simulink model "Generic_13"  (R2022b)
settings: Solver=VariableStepAuto  StartTime=0.0  StopTime=10.0  RelTol=1e-3
values from neighbouring files (symbols this model uses):
  A = cell2mat(A_cell)    [MPCController1.m]    (also in MPC_Fmincon.m)
  B = cell2mat(B_cell)    [MPCController1.m]    (also in MPC_Fmincon.m)
  brake_select = ones(length(speed), length(steering_angle))    [TwoDLook_uptable.m]
  curvature = 0.000:0.001:1    [TwoDLook_uptable.m]
  m = 1600    [MPCController1.m]    (also in MPCController2.m; MPC_Fmincon.m)
  speed = 0:0.1:100    [TwoDLook_uptable.m]
undefined symbols (not defined in the file or in its folder): Amplifier, DiscIntNeverNeededParam, K_d_yawrate, K_dsteering, k_speed, k_stanley, kd, ki, kp, path_curvature
libraries: CarMaker4SL x121, simulink x12, cstblocks x7, autolibshared x1, mpcadaslib x1
(part 4 of 5)

== matlab function Generic_13/CreateBus VhclCtrl/Stanley  steering & speed//Brake controller/Road sensor set & path planning/Road sensor set & path planning/Cross_track_error_calcuation/Cross_track_error_calcuation ==
  data: x_vehicle input; cte output; y_vehicle input; x_point input; y_point input; denominator output; x2 input; y2 input
function [cte,denominator]= calculate_cross_track_error(x_vehicle, y_vehicle, x_point, y_point,x2,y2)
    % Calculate cross-track error for a given vehicle position and single point
    function cte = calculate_perpendicular_distance(x_vehicle, y_vehicle, x_point, y_point)
    % Calculate the perpendicular distance from the vehicle to the point

    % Coordinates of the point
    x1 = x_point;
    y1 = y_point;
    %x2 = x_vehicle;
    %y2 = y_vehicle;

    % Calculate the cross-track error using the formula for the distance from a point to a line
    numerator = (x2 - x1) * (y1 - y_vehicle) - (x1 - x_vehicle) * (y2 - y1);
    denominator = sqrt((x2 - x1)^2 + (y2 - y1)^2);

    % Ensure that the denominator is not zero to avoid division by zero
    if denominator ~= 0
        cte = (numerator / denominator);
    else
        cte = 0;
    end
end
    % Calculate cross-track error as the perpendicular distance
    cte = calculate_perpendicular_distance(x_vehicle, y_vehicle, x_point, y_point);
end

== matlab function Generic_13/CreateBus VhclCtrl/Stanley  steering & speed//Brake controller/Road sensor set & path planning/Road sensor set & path planning/path_planning/Basic_obstacle avoidance ==
  data: Car_x input; updated_path output; Car_y input; dx input; dy input; object_width input; object_length input; path_x input; path_y input; car_v input; car_v_ceil input
function updated_path = obstacleAvoidanceSimulink(Car_x, Car_y, dx, dy, object_width, object_length, path_x, path_y,car_v, car_v_ceil)
    % Parameters
    if car_v >14
    safety_distance = car_v; % Adjust based on your requirements
    else
        safety_distance = 14;
    end
    %disp(car_v)
    % Check if the vehicle is close to the object
    distance_to_object = sqrt(dx^2 + dy^2);
    if (distance_to_object-object_length < safety_distance && distance_to_object > 0) && dx>0
        % Calculate the trajectory to avoid the entire obstacle
        angle_to_object = atan2(dy, dx);
        object_heading = atan2(object_length, object_width); % Assuming object is aligned with x-axis

        % Calculate new position to avoid the entire obstacle
        new_x = -1*(path_x + (car_v_ceil + object_length) * sin(angle_to_object + object_heading));
        new_y = -1*(path_y + (car_v_ceil + object_width/2) * cos(angle_to_object + object_heading));

        % Update the path to follow the new trajectory
        updated_path = [new_x; new_y] * ones(1, length(path_x));
    else
        updated_path = [path_x; path_y];
        %window_size = 5; % adjust the window size as needed
    %path_curvature = smoothdata(path_curvature, 'movmean', window_size)
    end
end

== matlab function Generic_13/CreateBus VhclCtrl/Stanley  steering & speed//Brake controller/Stanley_controller_with_thottle_and_brake_commands/MPCLongitudianl_contorl/MATLAB Function1 ==
  data: speed input; desired_speed output; distance_to_obstacle input; min_speed input
function desired_speed = advancedCollisionAvoidance(speed, distance_to_obstacle, min_speed)
    % Parameters
    max_acceleration = 3.0; % Maximum allowable acceleration
    max_deceleration = 5.0; % Maximum allowable deceleration
    prediction_horizon = 5; % Prediction horizon in seconds
    time_step = 0.1; % Time step for prediction
    safety_factor = 1.2; % Safety factor for braking distance estimation
    function braking_distance = calculateBrakingDistance(speed, max_deceleration, safety_factor)
    % Estimate the braking distance
    braking_distance = (speed^2) / (2 * max_deceleration) * safety_factor;
    end
    % Calculate the remaining braking distance
    braking_distance = calculateBrakingDistance(speed, max_deceleration, safety_factor);

    % Create a prediction model (simple linear model)
    A = 1; % State transition matrix
    B = -1; % Input matrix
    C = 1; % Output matrix
    Q = 1; % State cost
    R = 1; % Input cost
    N = 5; % Prediction horizon
    
    % Formulate the quadratic cost function
    H = blkdiag(2*(Q + R), repmat(2*Q, 1, N-1));
    
    % Constraints
    lb = min_speed * ones(N, 1);
    ub = speed * ones(N, 1) + max_acceleration * prediction_horizon * time_step;
    
    % Formulate the inequality constraints
    A_ineq = [eye(N); -eye(N)];
    b_ineq = [ub; -lb];
    
    % Initial guess (simple constant acceleration)
    u0 = ones(N, 1) * max_acceleration;
    
    % Solve the quadratic program
    options = optimoptions('quadprog', 'Display', 'off');
    u = quadprog(H, [], A_ineq, b_ineq, [], [], lb, ub, u0, options);
    
    % Apply the first control input as the desired acceleration
    desired_acceleration = u(1);
    
    % Adjust acceleration based on the distance to the obstacle and remaining braking distance
    if distance_to_obstacle < braking_distance
        % Apply maximum deceleration to stop before the obstacle
        desired_acceleration = -max_deceleration;
    end
    
    % Update the speed using the dynamics model
    desired_speed = speed + desired_acceleration * time_step;
    
    % Ensure the desired speed is within limits
    desired_speed = max(min_speed, min(desired_speed, speed + max_deceleration * time_step));
end

== matlab function Generic_13/CreateBus VhclCtrl/Stanley  steering & speed//Brake controller/Stanley_controller_with_thottle_and_brake_commands/MPCLongitudianl_contorl/Speed_regulator/Desired_speed_calc ==
  data: current_speed input; desired_speed output; distance_to_obstacle input; braking_distance input; relative_velocity input; speed_to_reach input; min_speed input; closing_velocity output; effective_distance output; safe_following_distance output
function [desired_speed,closing_velocity,effective_distance,safe_following_distance]= advancedCollisionAvoidance(current_speed, distance_to_obstacle,braking_distance, relative_velocity, speed_to_reach, min_speed)
    

    % Parameters
    max_deceleration = 5.0; % Maximum deceleration (adjust based on your requirements)
    reaction_time = 1.0; % Reaction time of the driver (adjust based on your requirements)
    % Calculate the remaining braking distance
    %braking_distance = calculateBrakingDistance(current_speed, max_deceleration, safety_factor);
    % Calculate the time required to stop the vehicle
    time_to_stop = current_speed / max_deceleration;

    % Calculate the required deceleration to stop before the obstacle
    required_deceleration = -current_speed / time_to_stop;

    % Calculate the projected distance the vehicle would cover during reaction time
    reaction_distance = current_speed * reaction_time;

    % Calculate the safe following distance based on reaction time and braking distance
    safe_following_distance = reaction_distance + braking_distance;

    % Calculate the effective distance to the obstacle considering reaction time
    effective_distance = distance_to_obstacle - reaction_distance;

    % Calculate the relative closing velocity
    closing_velocity = current_speed ;%- relative_velocity;

    % Determine if collision is imminent and adjust speed accordingly
    if (effective_distance < safe_following_distance-current_speed-5 && closing_velocity > 0)&& distance_to_obstacle ~=0
        % Apply maximum deceleration to avoid collision
        desired_speed = max(min_speed, current_speed + required_deceleration);
    elseif distance_to_obstacle>0 && distance_to_obstacle <5 && current_speed > 0
        desired_speed = 0;
    else
        desired_speed = speed_to_reach;
    end
end

== matlab function Generic_13/CreateBus VhclCtrl/Stanley  steering & speed//Brake controller/Stanley_controller_with_thottle_and_brake_commands/MPCLongitudianl_contorl/Speed_regulator/status_changing ==
  data: current_speed input; braking output; distance_to_obstacle input; relative_velocity input; steering_angle input; steering output; resume_driving output
function [braking, steering, resume_driving] = sophisticatedCollisionAvoidanceLogic(current_speed, distance_to_obstacle, relative_velocity, steering_angle)
   
    
    function braking_distance = calculateBrakingDistance(speed, max_deceleration, safety_factor)
        % Estimate the braking distance
        braking_distance = (speed^2) / (2 * max_deceleration) * safety_factor;
   end
   
% Parameters
    max_deceleration = 5.0; % Maximum deceleration (adjust based on your requirements)
    reaction_time = 1.0; % Reaction time of the driver (adjust based on your requirements)
    steering_threshold = 0; % Steering angle threshold to initiate steering (adjust based on your requirements)
    resume_distance = 15.0; % Distance at which the vehicle resumes normal driving after collision avoidance (adjust based on your requirements)
    safety_factor = 1.5;

    % Calculate the remaining braking distance
    braking_distance = calculateBrakingDistance(current_speed, max_deceleration, safety_factor);
    % Calculate the time required to stop the vehicle
    time_to_stop = current_speed / max_deceleration;

    % Calculate the projected distance the vehicle would cover during reaction time
    reaction_distance = current_speed * reaction_time;

    % Calculate the safe following distance based on reaction time and braking distance
    safe_following_distance = reaction_distance + braking_distance;

    % Calculate the effective distance to the obstacle considering reaction time
    effective_distance = distance_to_obstacle - reaction_distance;

    % Calculate the relative closing velocity
    closing_velocity = current_speed - relative_velocity;

    % Initialize braking, steering, and resume signals
    braking = 0;
    steering = 0;
    resume_driving = 0;

    % Collision avoidance logic
    if effective_distance < safe_following_distance && closing_velocity > 0
        % Apply maximum deceleration to avoid collision
        braking = 1;
    elseif abs(steering_angle) > steering_threshold
        % Apply steering if the steering angle is beyond a threshold
        steering = 1;
    elseif effective_distance > resume_distance
        % Resume normal driving if the obstacle is sufficiently far away
        resume_driving = 1;
    end
end

== matlab function Generic_13/CreateBus VhclCtrl/Stanley  steering & speed//Brake controller/Road sensor set & path planning/Road sensor set & path planning/Spline_path_planning/Spline_bsed_obstacle avoidance ==
  data: Car_x input; updated_path output; Car_y input; dx input; dy input; object_width input; object_length input; car_v input; pathx input; path_y input
function updated_path = obstacleAvoidanceWithSmoothPath(Car_x,Car_y, dx, dy, object_width, object_length, car_v, pathx, path_y)
    function generated_path = generateSmoothPath(control_points)
    % Parameters
    num_points = length(control_points);
    generated_path = zeros(2,41);
    % Ensure at least two control points are provided
    if num_points < 2
        error('At least two control points are required.');
    end
    
    % Extract x and y coordinates of control points
    x_points = zeros(1, num_points);
    y_points = zeros(1, num_points);
    
    for i = 1:num_points
        x_points(i) = control_points{i}(1);
        y_points(i) = control_points{i}(2);
    end
    
    % Generate a smooth path using spline interpolation
    t = 1:num_points;
    ts = 1:0.1:num_points; % Increase the resolution for a smoother path
    smooth_x = spline(t, x_points, ts);
    smooth_y = spline(t, y_points, ts);
    
    % Combine x and y coordinates into a path matrix
    generated_path = [smooth_x; smooth_y];
end

% Parameters
    if car_v > 14
        safety_distance = car_v; % Adjust based on your requirements
    else
        safety_distance = 14;
    end

    % Check if the vehicle is close to the object
    distance_to_object = sqrt(dx^2 + dy^2);
    if (distance_to_object - object_length < safety_distance && distance_to_object > 0) && dx > 0
        % Calculate the control points for generating a smooth path
        vehicle_point = [Car_x; Car_y];
        middle_point = [(Car_x + Car_x + dx) / 2; (Car_y + Car_y + dy) / 2];
        safe_point = [Car_x + dx - safety_distance; Car_y + dy];
        obstacle_point = [Car_x + dx + object_length; Car_y + dy+object_width/2];
        post_obstacle_point = [Car_x + dx + object_length + safety_distance; Car_y + dy];

        control_points = {vehicle_point, middle_point, safe_point, obstacle_point, post_obstacle_point};

        % Generate a smooth path using spline interpolation
        generated_path = generateSmoothPath(control_points);

        % Update the path to follow the generated smooth path
        updated_path = generated_path;
    else
        % If not close to the object, maintain the current path
        updated_path = [ones(1,41)*pathx; ones(1,41)*path_y];
    end
end

% Example usage
% Call this function with appropriate input arguments
% Ensure that you have the necessary parameters like Car_x, Car_y, dx, dy, etc.
% generated_path = obstacleAvoidanceWithSmoothPath(Car_x, Car_y, dx, dy, object_width, object_length, car_v, car_v_ceil);

== matlab function Generic_13/CreateBus VhclCtrl/Stanley  steering & speed//Brake controller/Stanley_controller_with_thottle_and_brake_commands/Stanley steering + PID speed controller/Speed_controller/advancedPID_speed_and_brake_control ==
  settings: updateMethod=DISCRETE
  data: path_curv input; throttle output; min_s_speed input; brake_cmd output; speed_act input; desired_speed input; Kd_speed input; Ki_speed input; Kp_speed input
function [throttle, brake_cmd] = advanced_speed_and_brake_control(path_curv, min_s_speed, speed_act, desired_speed,Kd_speed,Ki_speed,Kp_speed)
    persistent integrator_speed;
    persistent prev_speed_error;
    persistent integrator_brake;
    persistent prev_brake_error;

    if isempty(integrator_speed)
        integrator_speed = 0;
        prev_speed_error = 0;
        integrator_brake = 0;
        prev_brake_error = 0;
    end


   
    % Speed Control (PID)
    %disp(speed_act)
    %disp("teh speed is ")
    %disp(desired_speed)
    speed_error = desired_speed - speed_act;
    %Kp_speed = 1.900;
    %Ki_speed = 0.0300;
    %Kd_speed = 1.00;
    integrator_speed = integrator_speed + speed_error;
    derivative_speed = speed_error - prev_speed_error;
    
    throttle = Kp_speed * speed_error + Ki_speed * integrator_speed + Kd_speed * derivative_speed;

    % Braking Control (PID)
    brake_error = -speed_error;
    Kp_brake = 0.05;
    Ki_brake = 0.01;
    Kd_brake = 0.05;
    integrator_brake = integrator_brake + brake_error;
    derivative_brake = brake_error - prev_brake_error;
    brake_cmd = Kp_brake * brake_error + Ki_brake * integrator_brake + Kd_brake * derivative_brake;

    % Predictive Braking based on Path Curvature
    path_curvature = max(path_curv);
    min_safe_speed = max(min_s_speed);
    predictive_brake_factor = speed_act/100;
    if path_curvature > 0 && speed_act < min_safe_speed
        brake_cmd = brake_cmd + predictive_brake_factor * (min_safe_speed - speed_act);
    end
    % Update persistent variables
    prev_speed_error = speed_error;
    prev_brake_error = brake_error;
end

== matlab function Generic_13/CreateBus VhclCtrl/Stanley  steering & speed//Brake controller/Road sensor set & path planning/Road sensor set & path planning/Spline_path_planning/getInstantaneousPath Function ==
  data: generated_path input; lookahead_distance input; current_position input; instantaneous_points output; current_heading input
function instantaneous_points = getInstantaneousPoint(generated_path, lookahead_distance, current_position, current_heading)
    % Parameters
    num_points = size(generated_path, 2);
    rotated_point = zeros(1,2);
    instantaneous_point= zeros(1,2);
    disp(generated_path)
    % Find the closest point on the generated path to the current position
    distances = sqrt((generated_path(1, :) - current_position(1)).^2 + (generated_path(2, :) - current_position(2)).^2);
    [~, closest_point_index] = min(distances);
     % Extract the last point along the path based on lookahead distance
    cumulative_distances = cumsum(sqrt(diff(generated_path(1, :)).^2 + diff(generated_path(2, :)).^2));
     % Check if cumulative_distances is non-empty
    if all(cumulative_distances == 0)
        % If there is only one point in the path, use that point
        lookahead_index = closest_point_index;
    else
        % Otherwise, find the index based on lookahead distance
        lookahead_index = closest_point_index + find(cumulative_distances >= lookahead_distance, 1, 'first');
    end
    disp(lookahead_index)
    disp('333')
    
    % Ensure lookahead_index is within valid range
    lookahead_index = min(lookahead_index, num_points);
    
    % Extract the last point from the path
    instantaneous_point = generated_path(:, lookahead_index);
    
    % Transform the point to the vehicle's local coordinate system
    delta_x = instantaneous_point(1) - current_position(1);
    delta_y = instantaneous_point(2) - current_position(2);
    
    rotated_point = [cos(-current_heading) -sin(-current_heading); sin(-current_heading) cos(-current_heading)] * [delta_x; delta_y];
    
    % Adjust the rotated point to be relative to the current position
    instantaneous_points = [current_position(1) + rotated_point(1) current_position(2) + rotated_point(2)];
end

== matlab function Generic_13/CreateBus VhclCtrl/Stanley  steering & speed//Brake controller/Road sensor set & path planning/Road sensor set & path planning/Be'zeir path planning/Basic_obstacle avoidance ==
  data: initial_position input; updated_path output; final_position input; obstacle_width input; obstacle_length input; car_width input; car_length input; dx input; dy input; car_v input; path_x input; path_y input
function updated_path = obstacleAvoidanceWithPathPlanning(initial_position, final_position, obstacle_width, obstacle_length, car_width, car_length, dx, dy, car_v, path_x, path_y)
    function generated_path = generateObstacleFreeBezierPath(initial_position, final_position, obstacle_width, obstacle_length, car_width, obstacle_distance)
    % Calculate control points, obstacle position, and obstacle radius
    function control_points = calculateControlPoints(initial_position, final_position, obstacle_width, car_width, obstacle_distance)
        % Calculate control points for Bezier interpolation
        control_points = [
            initial_position;
            initial_position + [obstacle_distance/2; 0];
            initial_position + [obstacle_distance; obstacle_width/2];
            final_position - [obstacle_distance; obstacle_width/2];
            final_position - [obstacle_distance/2; 0];
            final_position
        ];
        
        % Adjust control points to ensure a smooth path
        control_points(3, 2) = control_points(1, 2) + car_width/2;
        control_points(4, 2) = control_points(6, 2) - car_width/2;
    end
    function obstacle_position = calculateObstaclePosition(initial_position, final_position, obstacle_distance)
        % Calculate obstacle position based on initial and final positions
        obstacle_position = (initial_position + final_position) / 2;
        obstacle_position(1) = obstacle_position(1) + obstacle_distance;
    end

    function result = bezierInterpolation(t, points)
            % Bezier interpolation function
            n = length(points) - 1;
            result = zeros(size(t));
            
            for i = 0:n
                result = result + nchoosek(n, i) * (1 - t).^(n - i) .* t.^i * points(i + 1);
            end
        end
        function collision = checkCollision(x, y, obstacle_position, obstacle_radius, resolution)
        % Collision checking function
        distances = sqrt((x - obstacle_position(1)).^2 + (y - obstacle_position(2)).^2);
        collision = any(distances <= obstacle_radius + resolution);
    end

    function adjusted_points = adjustControlPoints(control_points, obstacle_position, obstacle_radius, resolution)
        % Adjust control points to avoid the obstacle
        adjusted_points = control_points;
        
        % Find the control point closest to the obstacle
        distances = sqrt((control_points(1, :) - obstacle_position(1)).^2 + (control_points(2, :) - obstacle_position(2)).^2);
        [~, closest_point_index] = min(distances);
        disp(distances)
        % Move the closest control point away from the obstacle
        direction = (control_points(closest_point_index, :) - obstacle_position) / norm(control_points(closest_point_index,:) - obstacle_position);
        adjusted_points(closest_point_index,:) = obstacle_position + (obstacle_radius + resolution) * direction;
    end
    control_points = calculateControlPoints(initial_position, final_position, obstacle_width, car_width, obstacle_distance);
    obstacle_position = calculateObstaclePosition(initial_position, final_position, obstacle_distance);
    obstacle_radius = (obstacle_width + obstacle_length) / 4; % Assuming circular obstacle
    
    % Parameters
    num_points = size(control_points, 2);
    
    % Ensure at least two control points are provided
    if num_points < 2
        error('At least two control points are required.');
    end
    
    % Collision checking parameters
    collision_resolution = 0.1; % Resolution for collision checking
    
    % Extract x and y coordinates of control points
    x_points = control_points(1, :);
    y_points = control_points(2, :);
    
    % Bezier interpolation
    t = linspace(0, 1, num_points); % Parameter values
    Bx = bezierInterpolation(t, x_points);
    By = bezierInterpolation(t, y_points);
    
    % Check for collisions during interpolation
    % Check for collisions during interpolation using a while loop
    i = 1;
    while i <= length(Bx)
        if checkCollision(Bx(i), By(i), obstacle_position, obstacle_radius, collision_resolution)
            % Adjust the control points to avoid the obstacle
            control_points = adjustControlPoints(control_points, obstacle_position, obstacle_radius, collision_resolution);
            
            % Recalculate Bezier interpolation
            x_points = control_points(1, :);
            y_points = control_points(2, :);
            Bx = bezierInterpolation(t, x_points);
            By = bezierInterpolation(t, y_points);
            
            % Restart the collision checking loop
            i = 1;
        else
            % Increment the loop index if no collision
            i = i + 1;
        end
    end
    
    % Combine x and y coordinates into a path matrix
    generated_path = [Bx; By];
    end

    % Parameters
    if car_v > 14
        safety_distance = car_v; % Adjust based on your requirements
    else
        safety_distance = 14;
    end

    % Check if the vehicle is close to the object
    distance_to_object = sqrt(dx^2 + dy^2);
    obstacle_distance = distance_to_object;
    if (distance_to_object - obstacle_length < safety_distance && distance_to_object > 0) && dx > 0
        % Calculate the control points for generating a smooth path

        % Generate an obstacle-free path using Bezier interpolation
        generated_path = generateObstacleFreeBezierPath(initial_position, final_position, obstacle_width, obstacle_length, car_width, obstacle_distance);

        % Update the path to follow the generated obstacle-free path
        updated_path = generated_path;
    else
        % If not close to the object, maintain the current path
        updated_path = [ones(1,2)*path_x; ones(1,2)*path_y];
    end
end

== matlab function Generic_13/CreateBus VhclCtrl/Stanley  steering & speed//Brake controller/Road sensor set & path planning/Road sensor set & path planning/Be'zeir path planning/getInstantaneousPath Function ==
  data: generated_path input; lookahead_distance input; current_position input; instantaneous_points output; current_heading input
function instantaneous_points = getInstantaneousPoint(generated_path, lookahead_distance, current_position, current_heading)
    % Parameters
    num_points = size(generated_path, 2);
    rotated_point = zeros(1,2);
    instantaneous_point= zeros(1,2);
    disp(generated_path)
    % Find the closest point on the generated path to the current position
    distances = sqrt((generated_path(1, :) - current_position(1)).^2 + (generated_path(2, :) - current_position(2)).^2);
    [~, closest_point_index] = min(distances);
     % Extract the last point along the path based on lookahead distance
    cumulative_distances = cumsum(sqrt(diff(generated_path(1, :)).^2 + diff(generated_path(2, :)).^2));
     % Check if cumulative_distances is non-empty
    if all(cumulative_distances == 0)
        % If there is only one point in the path, use that point
        lookahead_index = closest_point_index;
    else
        % Otherwise, find the index based on lookahead distance
        lookahead_index = closest_point_index + find(cumulative_distances >= lookahead_distance, 1, 'first');
    end
    disp(lookahead_index)
    disp('333')
    
    % Ensure lookahead_index is within valid range
    lookahead_index = min(lookahead_index, num_points);
    
    % Extract the last point from the path
    instantaneous_point = generated_path(:, lookahead_index);
    
    % Transform the point to the vehicle's local coordinate system
    delta_x = instantaneous_point(1) - current_position(1);
    delta_y = instantaneous_point(2) - current_position(2);
    
    rotated_point = [cos(-current_heading) -sin(-current_heading); sin(-current_heading) cos(-current_heading)] * [delta_x; delta_y];
    
    % Adjust the rotated point to be relative to the current position
    instantaneous_points = [current_position(1) + rotated_point(1) current_position(2) + rotated_point(2)];
end

== matlab function Generic_13/CreateBus VhclCtrl/Stanley  steering & speed//Brake controller/Road sensor set & path planning/Road sensor set & path planning/Be'zeir path planning/MATLAB Function ==
  data: current_position input; initial_position output; heading input; dy input; dx input; path_length input; final_position output
function [initial_position, final_position] = calculateInitialFinalPositions(current_position, heading, dy, dx, path_length)
    % Calculate initial position (current position of the vehicle)
    initial_position = current_position;
    obstacle_distance = sqrt(dx^2+dy^2);
    % Calculate final position (position after the obstacle)
    final_position = current_position + [obstacle_distance * cos(heading); obstacle_distance * sin(heading)];

    % Ensure the final position is within a reasonable distance
    if norm(final_position - current_position) < obstacle_distance
        final_position = current_position + [obstacle_distance; 0];
    end

    % Ensure the final position is within a reasonable distance along the path
    if norm(final_position - current_position) > path_length
        final_position = current_position + path_length * [cos(heading); sin(heading)];
    end
end

== matlab function Generic_13/CreateBus VhclCtrl/Stanley  steering & speed//Brake controller/Road sensor set & path planning/Road sensor set & path planning/A* star path planning/Basic_obstacle avoidance ==
  data: Car_x input; updated_path output; Car_y input; dx input; dy input; object_length input; object_width input; car_v input; path_x input; path_y input
function updated_path = obstacleAvoidanceWithPathPlanningAStar(Car_x, Car_y, dx, dy, object_length, object_width, car_v, path_x, path_y)
    function grid = createGrid(obstacle_positions, grid_size)
        % Create a grid representation with obstacles
        
        % Initialize the grid with zeros
        grid = zeros(grid_size);
    
        % Place obstacles in the grid
        for i = 1:size(obstacle_positions, 1)
            obstacle_row = obstacle_positions(i, 1);
            obstacle_col = obstacle_positions(i, 2);
            
            % Check if the obstacle position is within the grid
            if obstacle_row >= 1 && obstacle_row <= grid_size(1) && ...
               obstacle_col >= 1 && obstacle_col <= grid_size(2)
                grid(obstacle_row, obstacle_col) = 1;
            else
                continue;
            end
        end
    end
    function path = AStarPathfinding(grid, start, goal)
    % A* Pathfinding Algorithm
    function [minRow, minCol] = findLowestFCost(openList, fCost)
        % Find the node with the lowest F cost in the open list
        [minF, idx] = min(fCost(openList > 0));
        [minRow, minCol] = ind2sub(size(openList), find(openList > 0, 1, 'first', idx));
    end
    function h = heuristic(node, goal)
        % Euclidean distance heuristic
        h = norm(node - goal);
    end
    function c = cost(currentRow, currentCol, neighborRow, neighborCol)
        % Cost function (can be customized based on specific requirements)
        c = norm([currentRow, currentCol] - [neighborRow, neighborCol]);
    end
    
    function withinBounds = isWithinBounds(row, col, numRows, numCols)
        % Check if the given coordinates are within the grid bounds
        withinBounds = (row >= 1 && row <= numRows) && (col >= 1 && col <= numCols);
    end
    
    function path = reconstructPath(start, goal, closedList)
        % Reconstruct the path from the closed list
        path = goal;
        currentRow = goal(1);
        currentCol = goal(2);
        
        while ~isequal([currentRow, currentCol], start)
            for move = [-1, 0; 1, 0; 0, -1; 0, 1; -1, -1; -1, 1; 1, -1; 1, 1]'
                neighborRow = currentRow + move(1);
                neighborCol = currentCol + move(2);
                
                if closedList(neighborRow, neighborCol)
                    path = [neighborRow, neighborCol; path];
                    currentRow = neighborRow;
                    currentCol = neighborCol;
                    break;
                end
            end
        end
    end

    % Define possible movements (up, down, left, right, and diagonals)
    movements = [
        -1,  0; % Up
         1,  0; % Down
         0, -1; % Left
         0,  1; % Right
        -1, -1; % Diagonal Up-Left
        -1,  1; % Diagonal Up-Right
         1, -1; % Diagonal Down-Left
         1,  1  % Diagonal Down-Right
    ];
    
    % Size of the grid
    [rows, cols] = size(grid);
    
    % Initialize open and closed lists
    openList = zeros(rows, cols);
    closedList = zeros(rows, cols);
    
    % Initialize the cost and heuristic maps
    gCost = Inf(rows, cols);
    hCost = Inf(rows, cols);
    
    % Initialize the starting node
    startRow = start(1);
    startCol = start(2);
    gCost(startRow, startCol) = 0;
    hCost(startRow, startCol) = heuristic(start, goal);
    
    % Main loop
    while true
        % Find the node with the lowest F cost in the open list
        [currentRow, currentCol] = findLowestFCost(openList, gCost + hCost);
        
        % Check if the goal is reached
        if isequal([currentRow, currentCol], goal)
            path = reconstructPath(start, goal, closedList);
            return;
        end
        
        % Move the current node from open to closed
        openList(currentRow, currentCol) = 0;
        closedList(currentRow, currentCol) = 1;
        
        % Expand neighbors
        for move = movements'
            neighborRow = currentRow + move(1);
            neighborCol = currentCol + move(2);
            
            % Check if the neighbor is within bounds and not an obstacle
            if isWithinBounds(neighborRow, neighborCol, rows, cols) && ~grid(neighborRow, neighborCol)
                % Calculate tentative G cost
                tentativeGCost = gCost(currentRow, currentCol) + cost(currentRow, currentCol, neighborRow, neighborCol);
                
                % Check if the neighbor is not in the closed list or has a lower G cost
                if ~closedList(neighborRow, neighborCol) || tentativeGCost < gCost(neighborRow, neighborCol)
                    % Update G and H costs
                    gCost(neighborRow, neighborCol) = tentativeGCost;
                    hCost(neighborRow, neighborCol) = heuristic([neighborRow, neighborCol], goal);
                    
                    % Add the neighbor to the open list if not already in it
                    if ~openList(neighborRow, neighborCol)
                        openList(neighborRow, neighborCol) = 1;
                    end
                end
            end
        end
    end
end
% Parameters
    if car_v > 14
        safety_distance = car_v; % Adjust based on your requirements
    else
        safety_distance = 14;
    end

    % Check if the vehicle is close to the object
    distance_to_object = sqrt(dx^2 + dy^2);
    if (distance_to_object - object_length < safety_distance && distance_to_object > 0) && dx > 0
        % Calculate the control points for generating a smooth path
        obstacle_point = [Car_x + dx + object_length, Car_y + dy + object_width/2];
        
        post_obstacle_point = [Car_x + dx + object_length + safety_distance; Car_y + dy+object_width];

        % Call A* pathfinding algorithm to generate an obstacle-free path
        start = round([Car_y; Car_x]); % Note: Flip y and x for A* coordinates
        goal = round(post_obstacle_point); % Note: Flip y and x for A* coordinates
        grid = createGrid(obstacle_point, [10, 10]);
        aStarPath = AStarPathfinding(grid, start, goal);

        % Update the path to follow the generated obstacle-free path
        updated_path = aStarPath';
    else
        % If not close to the object, maintain the current path
        updated_path = [path_x; path_y];
    end
end

== matlab function Generic_13/CreateBus VhclCtrl/Stanley  steering & speed//Brake controller/Road sensor set & path planning/Road sensor set & path planning/Dijkestra path planning/Basic_obstacle avoidance ==
  data: Car_x input; updated_path output; Car_y input; dx input; dy input; object_length input; object_width input; car_v input; path_x input; path_y input
function updated_path = obstacleAvoidanceWithPathPlanningAStar(Car_x, Car_y, dx, dy, object_length, object_width, car_v, path_x, path_y)
    function grid = createGrid(obstacle_positions, grid_size)
        % Create a grid representation with obstacles
        
        % Initialize the grid with zeros
        grid = zeros(grid_size);
    
        % Place obstacles in the grid
        for i = 1:size(obstacle_positions, 1)
            obstacle_row = obstacle_positions(i, 1);
            obstacle_col = obstacle_positions(i, 2);
            
            % Check if the obstacle position is within the grid
            if obstacle_row >= 1 && obstacle_row <= grid_size(1) && ...
               obstacle_col >= 1 && obstacle_col <= grid_size(2)
                grid(obstacle_row, obstacle_col) = 1;
            else
                continue;
            end
        end
    end
function path = DijkstraPathfinding(grid, start, goal)
    % Dijkstra Pathfinding Algorithm
    function withinBounds = isWithinBounds(row, col, numRows, numCols)
    % Check if the given coordinates are within the grid bounds
    withinBounds = (row >= 1 && row <= numRows) && (col >= 1 && col <= numCols);
end

function [minRow, minCol] = findMinDistanceNode(distance, visited)
    % Find the unvisited node with the minimum distance
    minDistance = Inf;
    [minRow, minCol] = deal(0, 0);

    [rows, cols] = size(distance);
    for i = 1:rows
        for j = 1:cols
            if ~visited(i, j) && distance(i, j) < minDistance
                minDistance = distance(i, j);
                minRow = i;
                minCol = j;
            end
        end
    end
end

function path = reconstructPath(start, goal, visited)
    % Reconstruct the path from the visited map
    path = goal;
    currentRow = goal(1);
    currentCol = goal(2);
    
    while ~isequal([currentRow, currentCol], start)
        for move = [-1, 0; 1, 0; 0, -1; 0, 1; -1, -1; -1, 1; 1, -1; 1, 1]'
            neighborRow = currentRow + move(1);
            neighborCol = currentCol + move(2);
            
            if isWithinBounds(neighborRow, neighborCol, size(visited, 1), size(visited, 2)) && visited(neighborRow, neighborCol)
                path = [neighborRow, neighborCol; path];
                currentRow = neighborRow;
                currentCol = neighborCol;
                break;
            end
        end
    end
end
    % Size of the grid
    [rows, cols] = size(grid);
    
    % Initialize the distance and visited maps
    distance = Inf(rows, cols);
    visited = zeros(rows, cols);
    
    % Define possible movements (up, down, left, right, and diagonals)
    movements = [
        -1,  0; % Up
         1,  0; % Down
         0, -1; % Left
         0,  1; % Right
        -1, -1; % Diagonal Up-Left
        -1,  1; % Diagonal Up-Right
         1, -1; % Diagonal Down-Left
         1,  1  % Diagonal Down-Right
    ];
    
    % Initialize the starting node
    startRow = start(1);
    startCol = start(2);
    distance(startRow, startCol) = 0;
    
    % Main loop
    while true
        % Find the node with the minimum distance among unvisited nodes
        [currentRow, currentCol] = findMinDistanceNode(distance, visited);
        
        % Check if the goal is reached
        if isequal([currentRow, currentCol], goal)
            path = reconstructPath(start, goal, visited);
            return;
        end
        
        % Mark the current node as visited
        visited(currentRow, currentCol) = 1;
        
        % Update distances to neighbors
        for move = movements'
            neighborRow = currentRow + move(1);
            neighborCol = currentCol + move(2);
            
            % Check if the neighbor is within bounds and not visited
            if isWithinBounds(neighborRow, neighborCol, rows, cols) && ~visited(neighborRow, neighborCol)
                % Calculate tentative distance
                tentativeDistance = distance(currentRow, currentCol) + grid(neighborRow, neighborCol);
                
                % Update distance if shorter
                if tentativeDistance < distance(neighborRow, neighborCol)
                    distance(neighborRow, neighborCol) = tentativeDistance;
                end
            end
        end
    end
end


% Parameters
    if car_v > 14
        safety_distance = car_v; % Adjust based on your requirements
    else
        safety_distance = 14;
    end

    % Check if the vehicle is close to the object
    distance_to_object = sqrt(dx^2 + dy^2);
    if (distance_to_object - object_length < safety_distance && distance_to_object > 0) && dx > 0
        % Calculate the control points for generating a smooth path
        obstacle_point = [Car_x + dx + object_length, Car_y + dy + object_width/2];
        
        post_obstacle_point = [Car_x + dx + object_length + safety_distance; Car_y + dy+object_width];

        % Call A* pathfinding algorithm to generate an obstacle-free path
        start = round([Car_y; Car_x]); % Note: Flip y and x for A* coordinates
        goal = round(post_obstacle_point); % Note: Flip y and x for A* coordinates
        grid = createGrid(obstacle_point, [10, 10]);
        DijkstraPath = DijkstraPathfinding(grid, start, goal);

        % Update the path to follow the generated obstacle-free path
        updated_path = DijkstraPath';
    else
        % If not close to the object, maintain the current path
        updated_path = [path_x; path_y];
    end
end

== matlab function Generic_13/CreateBus VhclCtrl/Stanley  steering & speed//Brake controller/Road sensor set & path planning/Road sensor set & path planning/A* star path planning/getInstantaneousPath Function ==
  data: generated_path input; lookahead_distance input; current_position input; instantaneous_points output; current_heading input
function instantaneous_points = getInstantaneousPoint(generated_path, lookahead_distance, current_position, current_heading)
    % Parameters
    num_points = size(generated_path, 2);
    rotated_point = zeros(1,2);
    instantaneous_point= zeros(1,2);
    disp(generated_path)
    % Find the closest point on the generated path to the current position
    distances = sqrt((generated_path(1, :) - current_position(1)).^2 + (generated_path(2, :) - current_position(2)).^2);
    [~, closest_point_index] = min(distances);
     % Extract the last point along the path based on lookahead distance
    cumulative_distances = cumsum(sqrt(diff(generated_path(1, :)).^2 + diff(generated_path(2, :)).^2));
     % Check if cumulative_distances is non-empty
    if all(cumulative_distances == 0)
        % If there is only one point in the path, use that point
        lookahead_index = closest_point_index;
    else
        % Otherwise, find the index based on lookahead distance
        lookahead_index = closest_point_index + find(cumulative_distances >= lookahead_distance, 1, 'first');
    end
    disp(lookahead_index)
    disp('333')
    
    % Ensure lookahead_index is within valid range
    lookahead_index = min(lookahead_index, num_points);
    
    % Extract the last point from the path
    instantaneous_point = generated_path(:, lookahead_index);
    
    % Transform the point to the vehicle's local coordinate system
    delta_x = instantaneous_point(1) - current_position(1);
    delta_y = instantaneous_point(2) - current_position(2);
    
    rotated_point = [cos(-current_heading) -sin(-current_heading); sin(-current_heading) cos(-current_heading)] * [delta_x; delta_y];
    
    % Adjust the rotated point to be relative to the current position
    instantaneous_points = [current_position(1) + rotated_point(1) current_position(2) + rotated_point(2)];
end

== matlab function Generic_13/CreateBus VhclCtrl/Stanley  steering & speed//Brake controller/Road sensor set & path planning/Road sensor set & path planning/Dijkestra path planning/getInstantaneousPath Function ==
  data: generated_path input; lookahead_distance input; current_position input; instantaneous_points output; current_heading input
function instantaneous_points = getInstantaneousPoint(generated_path, lookahead_distance, current_position, current_heading)
    % Parameters
    num_points = size(generated_path, 2);
    rotated_point = zeros(1,2);
    instantaneous_point= zeros(1,2);
    disp(generated_path)
    % Find the closest point on the generated path to the current position
    distances = sqrt((generated_path(1, :) - current_position(1)).^2 + (generated_path(2, :) - current_position(2)).^2);
    [~, closest_point_index] = min(distances);
     % Extract the last point along the path based on lookahead distance
    cumulative_distances = cumsum(sqrt(diff(generated_path(1, :)).^2 + diff(generated_path(2, :)).^2));
     % Check if cumulative_distances is non-empty
    if all(cumulative_distances == 0)
        % If there is only one point in the path, use that point
        lookahead_index = closest_point_index;
    else
        % Otherwise, find the index based on lookahead distance
        lookahead_index = closest_point_index + find(cumulative_distances >= lookahead_distance, 1, 'first');
    end
    disp(lookahead_index)
    disp('333')
    
    % Ensure lookahead_index is within valid range
    lookahead_index = min(lookahead_index, num_points);
    
    % Extract the last point from the path
    instantaneous_point = generated_path(:, lookahead_index);
    
    % Transform the point to the vehicle's local coordinate system
    delta_x = instantaneous_point(1) - current_position(1);
    delta_y = instantaneous_point(2) - current_position(2);
    
    rotated_point = [cos(-current_heading) -sin(-current_heading); sin(-current_heading) cos(-current_heading)] * [delta_x; delta_y];
    
    % Adjust the rotated point to be relative to the current position
    instantaneous_points = [current_position(1) + rotated_point(1) current_position(2) + rotated_point(2)];
end

== matlab function Generic_13/CreateBus VhclCtrl/Stanley  steering & speed//Brake controller/Stanley_controller_with_thottle_and_brake_commands/MPCLongitudianl_contorl/Speed_regulator/MATLAB Function ==
  data: speed input; braking_distance output; friction input; others output
function [braking_distance,others]= calculateBrakingDistance(speed,friction)
    % Estimate the braking distance
        max_deceleration = 5.0;
        safety_factor = 1.5;
        braking_distance = (speed^2) / (2 * max_deceleration) * safety_factor;
        others = speed^2 *3.6/(250*friction)* safety_factor*2.2;
end

== matlab function Generic_13/CreateBus VhclCtrl/Stanley  steering & speed//Brake controller/Stanley_controller_with_thottle_and_brake_commands/MPCLongitudianl_contorl/MPC_speed_control ==
  data: speed_error input; throttle_Brake output; A input; B input
function throttle_Brake = MPC_speed_control(speed_error,A,B)
    % Model Predictive Controller (MPC) for speed contol
    %speed_ref  = speed_rf+0.4;
    %speed_error= current_speed - speed_ref;
    % Define MPC parameters
    Ts = 0.1;  % Sampling time
    N = 10;    % Prediction horizon
    Q = 1;     % State weight
    R = 1;     % Input weight
    S = 0.1;   % Terminal state weight (integral term)
    
    % State-space model (simplified for illustration)
    %A = 0.8;
    %B = Ts;
    
    % Define cost and constraints for fmincon
    costFunction = @(u) (speed_error + B * u)' * Q * (speed_error + B * u) + u' * R * u + S * sum(u);
    Aeq = [];
    Beq = [];
    Aineq = [];
    Bineq = [];
    lb = 0; % Lower bound on throttle_Brake
    ub = 1;  % Upper bound on throttle_Brake
    
    % Steady-state error constraint
    Aineq = [Aineq; B];
    Bineq = [Bineq; -speed_error];
    
    % Initial guess
    u0 = 0;
    
    % Solve optimization problem
    options = optimoptions('fmincon', 'Display', 'off', 'Algorithm', 'sqp');
    u_opt = fmincon(costFunction, u0, Aineq, Bineq, Aeq, Beq, lb, ub, [], options);
    
    % Extract control input (throttle_Brake) from the optimization result
    throttle_Brake = u_opt;
end

== matlab function Generic_13/CreateBus VhclCtrl/Cross_track_error_calcuation/Cross_track_error_calcuation ==
  data: x_vehicle input; cte output; y_vehicle input; x_point input; y_point input; denominator output; x2 input; y2 input
function [cte,denominator]= calculate_cross_track_error(x_vehicle, y_vehicle, x_point, y_point,x2,y2)
    % Calculate cross-track error for a given vehicle position and single point
    function cte = calculate_perpendicular_distance(x_vehicle, y_vehicle, x_point, y_point)
    % Calculate the perpendicular distance from the vehicle to the point

    % Coordinates of the point
    x1 = x_point;
    y1 = y_point;
    %x2 = x_vehicle;
    %y2 = y_vehicle;

    % Calculate the cross-track error using the formula for the distance from a point to a line
    numerator = (x2 - x1) * (y1 - y_vehicle) - (x1 - x_vehicle) * (y2 - y1);
    denominator = sqrt((x2 - x1)^2 + (y2 - y1)^2);

    % Ensure that the denominator is not zero to avoid division by zero
    if denominator ~= 0
        cte = (numerator / denominator);
    else
        cte = 0;
    end
end
    % Calculate cross-track error as the perpendicular distance
    cte = calculate_perpendicular_distance(x_vehicle, y_vehicle, x_point, y_point);
end

== matlab function Generic_13/CreateBus VhclCtrl/calculate_cross_track_error/calculate_cross_track_error ==
  data: x_vehicle input; cte output; y_vehicle input; x_point input; y_point input; slope output; x2 input; y2 input
function [cte,slope]= calculate_cross_track_error(x_vehicle, y_vehicle, x_point, y_point,x2,y2)
    % Calculate cross-track error for a given vehicle position and single point
    function cte = calculate_perpendicular_distance(x_vehicle, y_vehicle, x_point, y_point)
    % Calculate the perpendicular distance from the vehicle to the point

    % Coordinates of the point
    x1 = x_point;
    y1 = y_point;
    %x2 = x_vehicle;
    %y2 = y_vehicle;
    slope =  atan((y2-y1)/(x2-x1));
    % Calculate the cross-track error using the formula for the distance from a point to a line
    numerator = (x2 - x1) * (y1 - y_vehicle) - (x1 - x_vehicle) * (y2 - y1);
    denominator = sqrt((x2 - x1)^2 + (y2 - y1)^2);

    % Ensure that the denominator is not zero to avoid division by zero
    if denominator ~= 0
        cte = (numerator / denominator);
    else
        cte = 0;
    end
end
    % Calculate cross-track error as the perpendicular distance
    cte = calculate_perpendicular_distance(x_vehicle, y_vehicle, x_point, y_point);
end
